simulink model "lab_3_and_4_block_diagrams"  (R2014b)
settings: Solver=ode23tb  StartTime=0.0  StopTime=200  RelTol=1e-3
values from neighbouring files (symbols this model uses):
  B1 = 20    [fcs_lab_05_model_01_test.m]
  B2 = 30    [fcs_lab_05_model_01_test.m]
  B3 = 30    [fcs_lab_05_model_01_test.m]
  C = 10    [fcs_lab_05_model_02_test.m]    (also in fcs_lab_05_model_03_test.m)
  K1 = 15    [fcs_lab_05_model_01_test.m]
  K2 = 15    [fcs_lab_05_model_01_test.m]
  L1 = 1    [fcs_lab_05_model_03_test.m]
  L2 = 1    [fcs_lab_05_model_03_test.m]
  M1 = 750    [fcs_lab_05_model_01_test.m]
  M2 = 750    [fcs_lab_05_model_01_test.m]
  R1 = 10    [fcs_lab_05_model_03_test.m]
  R2 = 10    [fcs_lab_05_model_03_test.m]
settings Model: Creator=faiq1  LastModifiedBy=Mashkoor Ahmed
settings DataIOCC: LimitDataPoints=off  SaveFormat=Dataset
settings OptimizationCC: UseDivisionForNetSlopeComputation=off  SimCompilerOptimization=off
settings DebuggingCC: SolverPrmCheckMsg=none  FrameProcessingCompatibilityMsg=error
settings HardwareCC: ProdBitPerPointer=64  ProdLargestAtomicFloat=Float  ProdIntDivRoundTo=Zero  ProdEndianess=LittleEndian  ProdWordSize=64  ProdHWDeviceType=Intel->x86-64 (Windows64)
settings ModelReferenceCC: PropagateSignalLabelsOutOfModel=on
settings RTWCC: RTWCompilerOptimization=off
settings ConfigComp: CovMetricSettings=dw  CovHtmlReporting=on  CovSaveCumulativeToWorkspaceVar=on  CovSaveSingleToWorkspaceVar=on  CovExternalEMLEnable=off

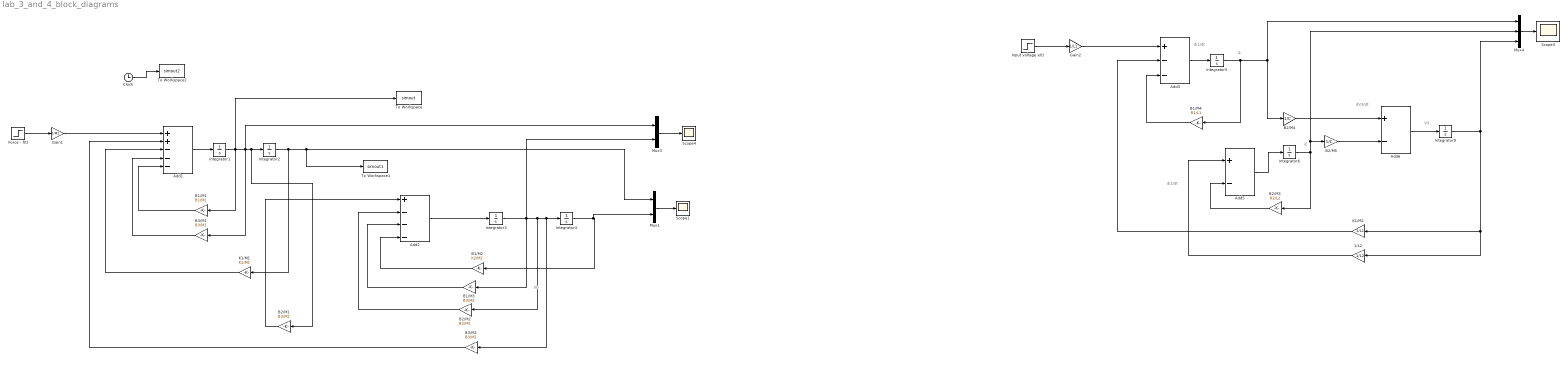
== system lab_3_and_4_block_diagrams ==
  note: di1/dt
  note: Xb
  note: i1
  note: i2
  note: V3
  note: dV3/dt
  note: di2/dt
  1/L2 : Gain  Gain=1/L2
  Add1 : Sum  Inputs=++---
  Add2 : Sum  Inputs=+---
  Add3 : Sum  Inputs=+--
  Add5 : Sum  Inputs=+-
  Add6 : Sum  Inputs=+-
  B1/M1 : Gain  Gain=B1/M1
  B1/M2 : Gain  Gain=K2/M2
  B1/M3 : Gain  Gain=B3/M2
  B1/M4 : Gain  Gain=R1/L1
  B2/M1 : Gain  Gain=B3/M2
  B2/M2 : Gain  Gain=B2/M2
  B2/M3 : Gain  Gain=R2/L2
  B2/M4 : Gain  Gain=1/C
  B2/M5 : Gain  Gain=1/C
  B3/M1 : Gain  Gain=B3/M1
  B3/M2 : Gain  Gain=B3/M1
  Clock : Clock
  Force - f(t) : Step  After=300  SampleTime=0
  Gain1 : Gain  Gain=1/M1
  Gain2 : Gain  Gain=1/L1
  Input voltage e(t) : Step  After=60  SampleTime=0
  Integrator{1..6,9} (7 alike) : Integrator
  K1/M1 : Gain  Gain=K1/M1
  K1/M2 : Gain  Gain=1/L1
  Mux1 : Mux  Inputs=2
  Mux3 : Mux  Inputs=2
  Mux4 : Mux  Inputs=3
  Scope1 : Scope
      settings: YMin=-5.00203  YMax=33.83101
  Scope3 : Scope
      settings: YMin=-3.68036  YMax=33.12327  SaveName=ScopeData3
  Scope4 : Scope
      settings: YMin=-1.56348  YMax=2.49523
  To Workspace : ToWorkspace  VariableName=simout  SaveFormat=Timeseries  SampleTime=-1
  To Workspace1 : ToWorkspace  VariableName=simout1  SaveFormat=Timeseries  SampleTime=-1
  To Workspace2 : ToWorkspace  VariableName=simout2  SaveFormat=Timeseries  SampleTime=-1
  wires:
  Add1/1 -> Integrator1/1
  Integrator1/1 -> B1/M1/1, Mux3/1, B3/M1/1, B2/M1/1, Integrator2/1, To Workspace/1
  Mux3/1 -> Scope4/1
  Integrator2/1 -> Mux1/1, To Workspace1/1, K1/M1/1
  B1/M1/1 -> Add1/5
  K1/M1/1 -> Add1/3
  Gain1/1 -> Add1/1
  Force - f(t)/1 -> Gain1/1
  Clock/1 -> To Workspace2/1
  B3/M1/1 -> Add1/4
  Add2/1 -> Integrator3/1
  Integrator4/1 -> Mux1/2, B1/M2/1
  B3/M2/1 -> Add1/2
  B1/M2/1 -> Add2/4
  B1/M3/1 -> Add2/3
  B2/M2/1 -> Add2/2
  B2/M1/1 -> Add2/1
  Integrator3/1 -> Mux3/2, B1/M3/1, B3/M2/1, Integrator4/1, B2/M2/1
  Mux1/1 -> Scope1/1
  Add3/1 -> Integrator5/1
  Integrator5/1 -> B2/M4/1, Mux4/1, B1/M4/1
  Mux4/1 -> Scope3/1
  Gain2/1 -> Add3/1
  Input voltage e(t)/1 -> Gain2/1
  Add5/1 -> Integrator6/1
  Integrator6/1 -> B2/M5/1, Mux4/2, B2/M3/1
  B2/M3/1 -> Add5/2
  Add6/1 -> Integrator9/1
  B2/M4/1 -> Add6/1
  B2/M5/1 -> Add6/2
  Integrator9/1 -> Mux4/3, 1/L2/1, K1/M2/1
  1/L2/1 -> Add5/1
  K1/M2/1 -> Add3/2
  B1/M4/1 -> Add3/3
